simulink model "Pendulum_Native_1"  (R2021a)
settings: Solver=FixedStepDiscrete  StartTime=0.0  StopTime=inf  FixedStep=0.01  RelTol=1e-3
PostLoadFcn:
  | addpath(fileparts(get_param('Pendulum_Native_1','FileName')),fullfile(fileparts(get_param('Pendulum_Native_1','FileName')),'..','hardware'));
InitFcn:
  | addpath(fileparts(get_param('Pendulum_Native_1','FileName')),fullfile(fileparts(get_param('Pendulum_Native_1','FileName')),'..','hardware'));
libraries: sldrtlib x1
settings Model: Creator=YW  LastModifiedBy=YW
settings DataIOCC: SaveOutput=off  SignalLogging=off  SaveTime=off
settings DebuggingCC: AlgebraicLoopMsg=error

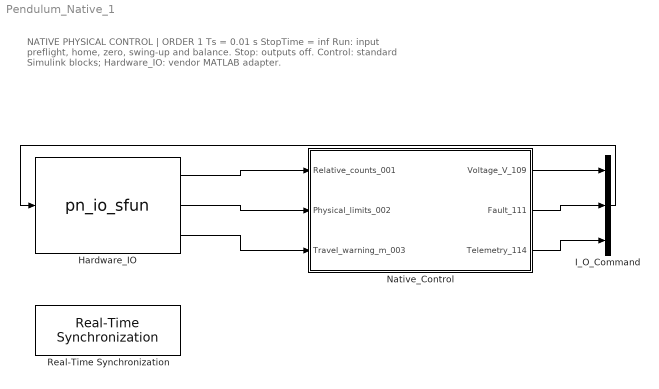
== system Pendulum_Native_1 ==
  note: NATIVE PHYSICAL CONTROL | ORDER 1
      | Ts = 0.01 s    StopTime = inf
      | Run: input preflight, home, zero, swing-up and balance. Stop: outputs off.
      | Control: standard Simulink blocks; Hardware_IO: vendor MATLAB adapter.
  Hardware_IO : M-S-Function  FunctionName=pn_io_sfun  Parameters=1
  I_O_Command : Mux  Inputs=3
  Native_Control : Subsystem
  Real-Time Synchronization : sldrtlib/Real-Time Synchronization  Priority=-100  SampleTime=0.01  MaxMissedTicks=1000000  ShowMissedTicks=off  YieldWhenWaiting=off
  wires:
  Hardware_IO/1 -> Native_Control/1(Relative_counts_001)
  Hardware_IO/2 -> Native_Control/2(Physical_limits_002)
  Hardware_IO/3 -> Native_Control/3(Travel_warning_m_003)
  Native_Control/1(Voltage_V_109) -> I_O_Command/1
  Native_Control/2(Fault_111) -> I_O_Command/2
  Native_Control/3(Telemetry_114) -> I_O_Command/3
  I_O_Command/1 -> Hardware_IO/1

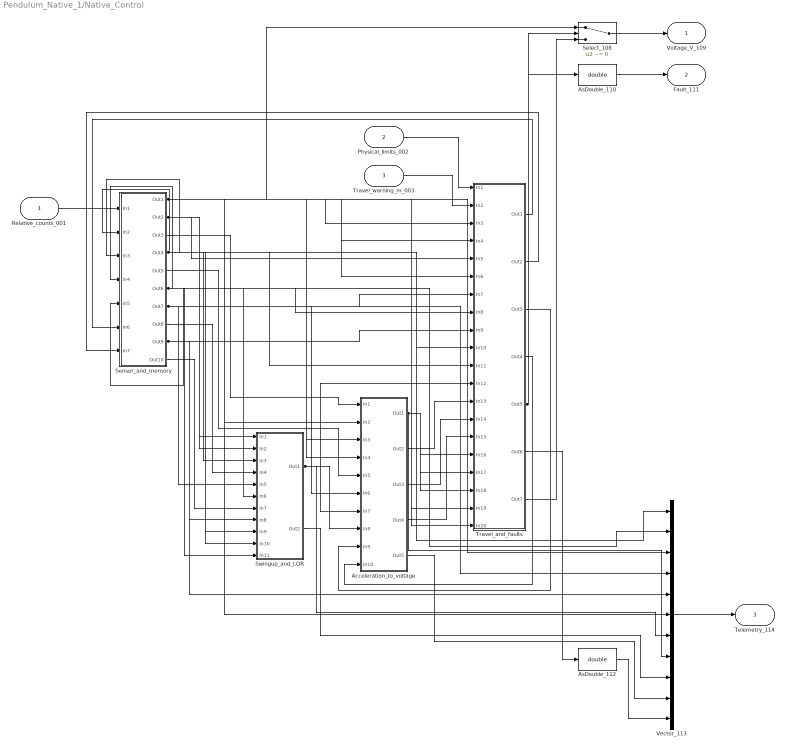
== system Pendulum_Native_1/Native_Control ==
  Relative_counts_001 : Inport  PortDimensions=2
  Physical_limits_002 : Inport  Port=2  PortDimensions=2
  Travel_warning_m_003 : Inport  Port=3  PortDimensions=1
  Acceleration_to_voltage : Subsystem
  AsDouble_110 : DataTypeConversion  OutDataTypeStr=double
  AsDouble_112 : DataTypeConversion  OutDataTypeStr=double
  Select_108 : Switch  Criteria=u2 ~= 0
  Sensor_and_memory : Subsystem
  Swingup_and_LQR : Subsystem
  Travel_and_faults : Subsystem
  Vector_113 : Mux  Inputs=11
  Voltage_V_109 : Outport
  Fault_111 : Outport  Port=2
  Telemetry_114 : Outport  Port=3
  wires:
  Travel_and_faults/4(Out4) -> Acceleration_to_voltage/10(In10)
  Vector_113/1 -> Telemetry_114/1
  Travel_and_faults/7(Out7) -> Select_108/3
  Travel_and_faults/3(Out3) -> Acceleration_to_voltage/9(In9)
  Travel_and_faults/6(Out6) -> AsDouble_112/1
  Travel_and_faults/2(Out2) -> Sensor_and_memory/7(In7)
  Travel_and_faults/1(Out1) -> Sensor_and_memory/6(In6)
  Sensor_and_memory/2(Out2) -> Travel_and_faults/5(In5), Swingup_and_LQR/1(In1), Swingup_and_LQR/2(In2)
  Acceleration_to_voltage/4(Out4) -> Travel_and_faults/15(In15)
  Select_108/1 -> Voltage_V_109/1
  Acceleration_to_voltage/3(Out3) -> Travel_and_faults/14(In14)
  Sensor_and_memory/5(Out5) -> Acceleration_to_voltage/5(In5)
  Acceleration_to_voltage/2(Out2) -> Travel_and_faults/13(In13)
  Sensor_and_memory/3(Out3) -> Acceleration_to_voltage/1(In1)
  Travel_warning_m_003/1 -> Travel_and_faults/2(In2)
  Sensor_and_memory/7(Out7) -> Vector_113/4, Acceleration_to_voltage/6(In6), Travel_and_faults/7(In7), Swingup_and_LQR/5(In5)
  Acceleration_to_voltage/1(Out1) -> Travel_and_faults/18(In18), Vector_113/8, Travel_and_faults/16(In16), Travel_and_faults/17(In17)
  Physical_limits_002/1 -> Travel_and_faults/1(In1)
  Acceleration_to_voltage/5(Out5) -> Vector_113/10
  Swingup_and_LQR/2(Out2) -> Vector_113/9
  Relative_counts_001/1 -> Sensor_and_memory/1(In1)
  Sensor_and_memory/10(Out10) -> Swingup_and_LQR/7(In7)
  Sensor_and_memory/8(Out8) -> Swingup_and_LQR/4(In4)
  AsDouble_112/1 -> Vector_113/11
  AsDouble_110/1 -> Fault_111/1
  Travel_and_faults/5(Out5) -> Select_108/2, AsDouble_110/1
  Swingup_and_LQR/1(Out1) -> Vector_113/7, Acceleration_to_voltage/7(In7), Acceleration_to_voltage/8(In8), Travel_and_faults/12(In12)
  Sensor_and_memory/1(Out1) -> Vector_113/3, Vector_113/6, Travel_and_faults/20(In20), Acceleration_to_voltage/3(In3), Select_108/1, Travel_and_faults/19(In19), Acceleration_to_voltage/4(In4), Travel_and_faults/6(In6), Acceleration_to_voltage/2(In2), Travel_and_faults/3(In3), Travel_and_faults/4(In4)
  Sensor_and_memory/4(Out4) -> Swingup_and_LQR/10(In10), Travel_and_faults/10(In10), Swingup_and_LQR/9(In9), Travel_and_faults/11(In11), Sensor_and_memory/3(In3), Vector_113/1, Sensor_and_memory/2(In2), Swingup_and_LQR/3(In3)
  Sensor_and_memory/6(Out6) -> Swingup_and_LQR/6(In6), Travel_and_faults/8(In8), Sensor_and_memory/4(In4), Swingup_and_LQR/11(In11), Vector_113/2, Sensor_and_memory/5(In5)
  Sensor_and_memory/9(Out9) -> Swingup_and_LQR/8(In8), Travel_and_faults/9(In9), Vector_113/5

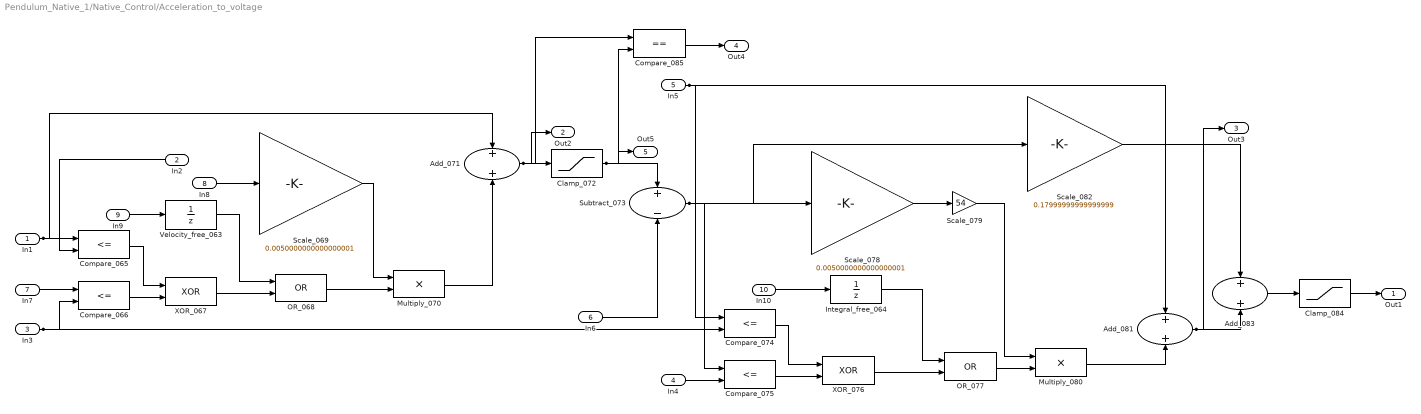
== system Pendulum_Native_1/Native_Control/Acceleration_to_voltage ==
  In1 : Inport
  In2 : Inport  Port=2
  In3 : Inport  Port=3
  In4 : Inport  Port=4
  In5 : Inport  Port=5
  In6 : Inport  Port=6
  In7 : Inport  Port=7
  In8 : Inport  Port=8
  In9 : Inport  Port=9
  In10 : Inport  Port=10
  Add_071 : Sum
  Add_081 : Sum
  Add_083 : Sum
  Clamp_072 : Saturate  UpperLimit=0.59999999999999998  LowerLimit=-0.59999999999999998
  Clamp_084 : Saturate  UpperLimit=1  LowerLimit=-1
  Compare_065 : RelationalOperator  Operator=<=  OutDataTypeStr=boolean  RndMeth=Simplest
  Compare_066 : RelationalOperator  Operator=<=  OutDataTypeStr=boolean  RndMeth=Simplest
  Compare_074 : RelationalOperator  Operator=<=  OutDataTypeStr=boolean  RndMeth=Simplest
  Compare_075 : RelationalOperator  Operator=<=  OutDataTypeStr=boolean  RndMeth=Simplest
  Compare_085 : RelationalOperator  Operator===  OutDataTypeStr=boolean  RndMeth=Simplest
  Integral_free_064 : UnitDelay  SampleTime=-1  HasFrameUpgradeWarning=on
  Multiply_070 : Product
  Multiply_080 : Product
  OR_068 : Logic  Operator=OR  AllPortsSameDT=off  OutDataTypeStr=boolean
  OR_077 : Logic  Operator=OR  AllPortsSameDT=off  OutDataTypeStr=boolean
  Scale_069 : Gain  Gain=0.0050000000000000001
  Scale_078 : Gain  Gain=0.0050000000000000001
  Scale_079 : Gain  Gain=54
  Scale_082 : Gain  Gain=0.17999999999999999
  Subtract_073 : Sum  Inputs=+-
  Velocity_free_063 : UnitDelay  SampleTime=-1  HasFrameUpgradeWarning=on
  XOR_067 : Logic  Operator=XOR  AllPortsSameDT=off  OutDataTypeStr=boolean
  XOR_076 : Logic  Operator=XOR  AllPortsSameDT=off  OutDataTypeStr=boolean
  Out1 : Outport
  Out2 : Outport  Port=2
  Out3 : Outport  Port=3
  Out4 : Outport  Port=4
  Out5 : Outport  Port=5
  wires:
  In6/1 -> Subtract_073/2
  In9/1 -> Velocity_free_063/1
  Compare_085/1 -> Out4/1
  In8/1 -> Scale_069/1
  In10/1 -> Integral_free_064/1
  Add_083/1 -> Clamp_084/1
  Scale_078/1 -> Scale_079/1
  Subtract_073/1 -> Compare_075/1, Scale_078/1, Scale_082/1
  OR_077/1 -> Multiply_080/2
  XOR_076/1 -> OR_077/2
  XOR_067/1 -> OR_068/2
  Scale_079/1 -> Multiply_080/1
  OR_068/1 -> Multiply_070/2
  In7/1 -> Compare_066/1
  In1/1 -> Add_071/1, Compare_065/1
  Compare_074/1 -> XOR_076/1
  Integral_free_064/1 -> OR_077/1
  Clamp_084/1 -> Out1/1
  Scale_069/1 -> Multiply_070/1
  Velocity_free_063/1 -> OR_068/1
  Multiply_070/1 -> Add_071/2
  Scale_082/1 -> Add_083/1
  Compare_066/1 -> XOR_067/2
  Multiply_080/1 -> Add_081/2
  Compare_075/1 -> XOR_076/2
  In2/1 -> Compare_065/2
  In4/1 -> Compare_075/2
  Compare_065/1 -> XOR_067/1
  Add_071/1 -> Compare_085/1, Out2/1, Clamp_072/1
  In3/1 -> Compare_066/2, Compare_074/2
  Clamp_072/1 -> Compare_085/2, Out5/1, Subtract_073/1
  Add_081/1 -> Add_083/2, Out3/1
  In5/1 -> Compare_074/1, Add_081/1

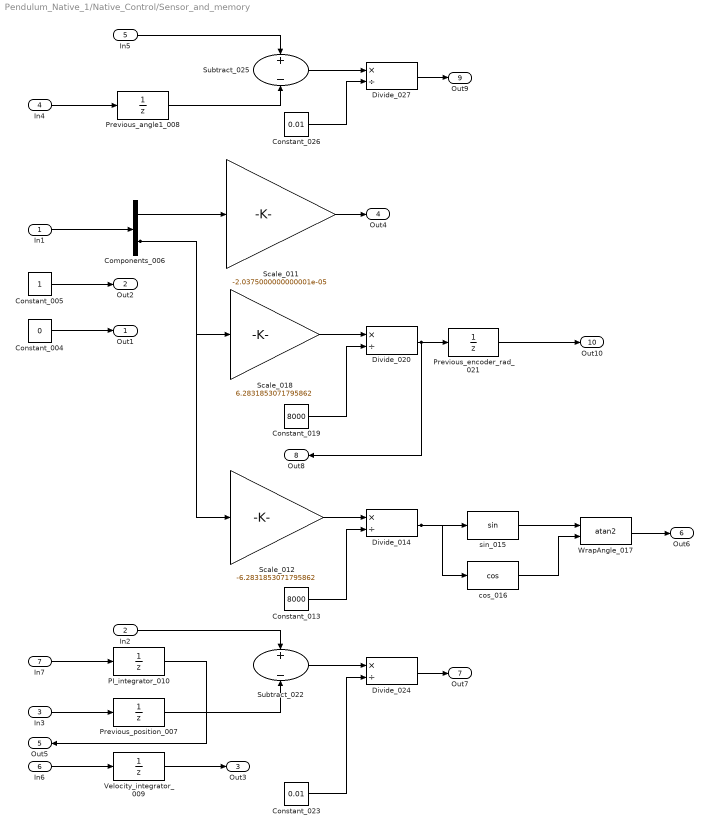
== system Pendulum_Native_1/Native_Control/Sensor_and_memory ==
  In1 : Inport
  In2 : Inport  Port=2
  In3 : Inport  Port=3
  In4 : Inport  Port=4
  In5 : Inport  Port=5
  In6 : Inport  Port=6
  In7 : Inport  Port=7
  Components_006 : Demux  Outputs=2
  Constant_004 : Constant  Value=0
  Constant_005 : Constant
  Constant_013 : Constant  Value=8000
  Constant_019 : Constant  Value=8000
  Constant_023 : Constant  Value=0.01
  Constant_026 : Constant  Value=0.01
  Divide_014 : Product  Inputs=*/
  Divide_020 : Product  Inputs=*/
  Divide_024 : Product  Inputs=*/
  Divide_027 : Product  Inputs=*/
  PI_integrator_010 : UnitDelay  SampleTime=-1  HasFrameUpgradeWarning=on
  Previous_angle1_008 : UnitDelay  SampleTime=-1  HasFrameUpgradeWarning=on
  Previous_encoder_rad_021 : UnitDelay  SampleTime=-1  HasFrameUpgradeWarning=on
  Previous_position_007 : UnitDelay  SampleTime=-1  HasFrameUpgradeWarning=on
  Scale_011 : Gain  Gain=-2.0375000000000001e-05
  Scale_012 : Gain  Gain=-6.2831853071795862
  Scale_018 : Gain  Gain=6.2831853071795862
  Subtract_022 : Sum  Inputs=+-
  Subtract_025 : Sum  Inputs=+-
  Velocity_integrator_009 : UnitDelay  SampleTime=-1  HasFrameUpgradeWarning=on
  WrapAngle_017 : Trigonometry  Operator=atan2
  cos_016 : Trigonometry  Operator=cos
  sin_015 : Trigonometry
  Out1 : Outport
  Out2 : Outport  Port=2
  Out3 : Outport  Port=3
  Out4 : Outport  Port=4
  Out5 : Outport  Port=5
  Out6 : Outport  Port=6
  Out7 : Outport  Port=7
  Out8 : Outport  Port=8
  Out9 : Outport  Port=9
  Out10 : Outport  Port=10
  wires:
  In5/1 -> Subtract_025/1
  In7/1 -> PI_integrator_010/1
  In4/1 -> Previous_angle1_008/1
  Scale_011/1 -> Out4/1
  PI_integrator_010/1 -> Out5/1
  Velocity_integrator_009/1 -> Out3/1
  Divide_024/1 -> Out7/1
  In3/1 -> Previous_position_007/1
  Divide_027/1 -> Out9/1
  Constant_004/1 -> Out1/1
  In1/1 -> Components_006/1
  Constant_026/1 -> Divide_027/2
  WrapAngle_017/1 -> Out6/1
  Scale_018/1 -> Divide_020/1
  Subtract_025/1 -> Divide_027/1
  In2/1 -> Subtract_022/1
  In6/1 -> Velocity_integrator_009/1
  Previous_position_007/1 -> Subtract_022/2
  Previous_encoder_rad_021/1 -> Out10/1
  Subtract_022/1 -> Divide_024/1
  Previous_angle1_008/1 -> Subtract_025/2
  Scale_012/1 -> Divide_014/1
  Constant_019/1 -> Divide_020/2
  sin_015/1 -> WrapAngle_017/1
  cos_016/1 -> WrapAngle_017/2
  Components_006/1 -> Scale_011/1
  Constant_023/1 -> Divide_024/2
  Constant_013/1 -> Divide_014/2
  Constant_005/1 -> Out2/1
  Divide_014/1 -> sin_015/1, cos_016/1
  Components_006/2 -> Scale_012/1, Scale_018/1
  Divide_020/1 -> Previous_encoder_rad_021/1, Out8/1

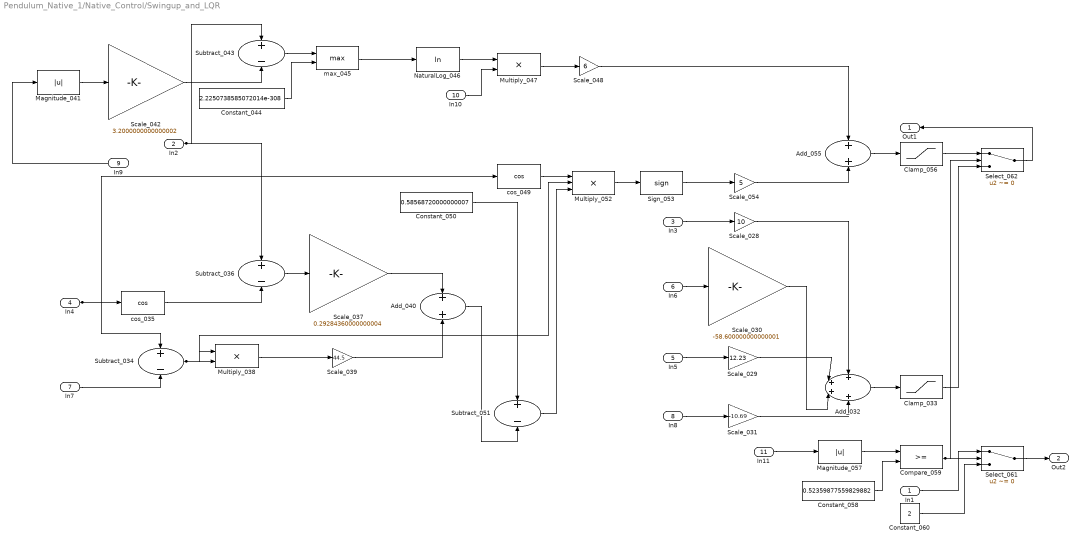
== system Pendulum_Native_1/Native_Control/Swingup_and_LQR ==
  In1 : Inport
  In2 : Inport  Port=2
  In3 : Inport  Port=3
  In4 : Inport  Port=4
  In5 : Inport  Port=5
  In6 : Inport  Port=6
  In7 : Inport  Port=7
  In8 : Inport  Port=8
  In9 : Inport  Port=9
  In10 : Inport  Port=10
  In11 : Inport  Port=11
  Add_032 : Sum  Inputs=++++
  Add_040 : Sum
  Add_055 : Sum
  Clamp_033 : Saturate  UpperLimit=10  LowerLimit=-10
  Clamp_056 : Saturate  UpperLimit=10  LowerLimit=-10
  Compare_059 : RelationalOperator  OutDataTypeStr=boolean  RndMeth=Simplest
  Constant_044 : Constant  Value=2.2250738585072014e-308
  Constant_050 : Constant  Value=0.58568720000000007
  Constant_058 : Constant  Value=0.52359877559829882
  Constant_060 : Constant  Value=2
  Magnitude_041 : Abs
  Magnitude_057 : Abs
  Multiply_038 : Product
  Multiply_047 : Product
  Multiply_052 : Product  Inputs=3
  NaturalLog_046 : Math  Operator=log  SaturateOnIntegerOverflow=on
  Scale_028 : Gain  Gain=10
  Scale_029 : Gain  Gain=12.23
  Scale_030 : Gain  Gain=-58.600000000000001
  Scale_031 : Gain  Gain=-10.69
  Scale_037 : Gain  Gain=0.29284360000000004
  Scale_039 : Gain  Gain=44.5
  Scale_042 : Gain  Gain=3.2000000000000002
  Scale_048 : Gain  Gain=6
  Scale_054 : Gain  Gain=5
  Select_061 : Switch  Criteria=u2 ~= 0
  Select_062 : Switch  Criteria=u2 ~= 0
  Sign_053 : Signum
  Subtract_034 : Sum  Inputs=+-
  Subtract_036 : Sum  Inputs=+-
  Subtract_043 : Sum  Inputs=+-
  Subtract_051 : Sum  Inputs=+-
  cos_035 : Trigonometry  Operator=cos
  cos_049 : Trigonometry  Operator=cos
  max_045 : MinMax  Function=max  Inputs=2
  Out1 : Outport
  Out2 : Outport  Port=2
  wires:
  In9/1 -> Magnitude_041/1
  Scale_054/1 -> Add_055/2
  In7/1 -> Subtract_034/2
  Select_062/1 -> Out1/1
  cos_049/1 -> Multiply_052/1
  Multiply_038/1 -> Scale_039/1
  Compare_059/1 -> Select_061/2, Select_062/2
  In10/1 -> Multiply_047/2
  In3/1 -> Scale_028/1
  In5/1 -> Scale_029/1
  Scale_029/1 -> Add_032/2
  In8/1 -> Scale_031/1
  In11/1 -> Magnitude_057/1
  NaturalLog_046/1 -> Multiply_047/1
  In6/1 -> Scale_030/1
  Multiply_047/1 -> Scale_048/1
  Subtract_043/1 -> max_045/1
  Sign_053/1 -> Scale_054/1
  Scale_028/1 -> Add_032/1
  Scale_042/1 -> Subtract_043/2
  Scale_039/1 -> Add_040/2
  Magnitude_057/1 -> Compare_059/1
  Magnitude_041/1 -> Scale_042/1
  Scale_031/1 -> Add_032/4
  Clamp_056/1 -> Select_062/1
  Constant_058/1 -> Compare_059/2
  Scale_037/1 -> Add_040/1
  Subtract_034/1 -> Multiply_038/2, Multiply_052/2, Multiply_038/1
  Scale_030/1 -> Add_032/3
  Add_032/1 -> Clamp_033/1
  Add_040/1 -> Subtract_051/2
  Subtract_036/1 -> Scale_037/1
  max_045/1 -> NaturalLog_046/1
  Add_055/1 -> Clamp_056/1
  Constant_050/1 -> Subtract_051/1
  Scale_048/1 -> Add_055/1
  Subtract_051/1 -> Multiply_052/3
  Constant_044/1 -> max_045/2
  Clamp_033/1 -> Select_062/3
  Constant_060/1 -> Select_061/3
  Multiply_052/1 -> Sign_053/1
  cos_035/1 -> Subtract_036/2
  In1/1 -> Select_061/1
  Select_061/1 -> Out2/1
  In2/1 -> Subtract_036/1, Subtract_043/1
  In4/1 -> cos_049/1, Subtract_034/1, cos_035/1

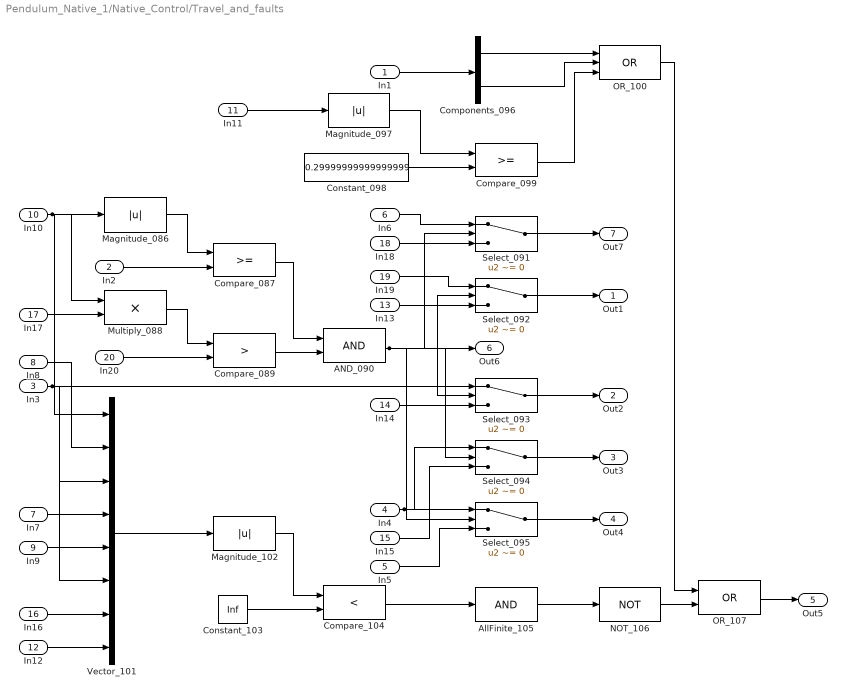
== system Pendulum_Native_1/Native_Control/Travel_and_faults ==
  In1 : Inport
  In2 : Inport  Port=2
  In3 : Inport  Port=3
  In4 : Inport  Port=4
  In5 : Inport  Port=5
  In6 : Inport  Port=6
  In7 : Inport  Port=7
  In8 : Inport  Port=8
  In9 : Inport  Port=9
  In10 : Inport  Port=10
  In11 : Inport  Port=11
  In12 : Inport  Port=12
  In13 : Inport  Port=13
  In14 : Inport  Port=14
  In15 : Inport  Port=15
  In16 : Inport  Port=16
  In17 : Inport  Port=17
  In18 : Inport  Port=18
  In19 : Inport  Port=19
  In20 : Inport  Port=20
  AND_090 : Logic  AllPortsSameDT=off  OutDataTypeStr=boolean
  AllFinite_105 : Logic  Inputs=1  AllPortsSameDT=off  OutDataTypeStr=boolean
  Compare_087 : RelationalOperator  OutDataTypeStr=boolean  RndMeth=Simplest
  Compare_089 : RelationalOperator  Operator=>  OutDataTypeStr=boolean  RndMeth=Simplest
  Compare_099 : RelationalOperator  OutDataTypeStr=boolean  RndMeth=Simplest
  Compare_104 : RelationalOperator  Operator=<  OutDataTypeStr=boolean  RndMeth=Simplest
  Components_096 : Demux  Outputs=2
  Constant_098 : Constant  Value=0.29999999999999999
  Constant_103 : Constant  Value=Inf
  Magnitude_086 : Abs
  Magnitude_097 : Abs
  Magnitude_102 : Abs
  Multiply_088 : Product
  NOT_106 : Logic  Operator=NOT  Inputs=1  AllPortsSameDT=off  OutDataTypeStr=boolean
  OR_100 : Logic  Operator=OR  Inputs=3  AllPortsSameDT=off  OutDataTypeStr=boolean
  OR_107 : Logic  Operator=OR  AllPortsSameDT=off  OutDataTypeStr=boolean
  Select_091 : Switch  Criteria=u2 ~= 0
  Select_092 : Switch  Criteria=u2 ~= 0
  Select_093 : Switch  Criteria=u2 ~= 0
  Select_094 : Switch  Criteria=u2 ~= 0
  Select_095 : Switch  Criteria=u2 ~= 0
  Vector_101 : Mux  Inputs=8
  Out1 : Outport
  Out2 : Outport  Port=2
  Out3 : Outport  Port=3
  Out4 : Outport  Port=4
  Out5 : Outport  Port=5
  Out6 : Outport  Port=6
  Out7 : Outport  Port=7
  wires:
  In8/1 -> Vector_101/2
  In20/1 -> Compare_089/2
  In2/1 -> Compare_087/2
  In16/1 -> Vector_101/7
  In7/1 -> Vector_101/4
  Constant_098/1 -> Compare_099/2
  In1/1 -> Components_096/1
  In17/1 -> Multiply_088/2
  Select_094/1 -> Out3/1
  In5/1 -> Select_095/3
  In15/1 -> Select_094/3
  Select_092/1 -> Out1/1
  In11/1 -> Magnitude_097/1
  Select_091/1 -> Out7/1
  Vector_101/1 -> Magnitude_102/1
  Constant_103/1 -> Compare_104/2
  AllFinite_105/1 -> NOT_106/1
  In9/1 -> Vector_101/5
  Components_096/1 -> OR_100/1
  Compare_099/1 -> OR_100/3
  In14/1 -> Select_093/3
  NOT_106/1 -> OR_107/2
  Magnitude_097/1 -> Compare_099/1
  In12/1 -> Vector_101/8
  Magnitude_086/1 -> Compare_087/1
  In13/1 -> Select_092/3
  Select_095/1 -> Out4/1
  In19/1 -> Select_092/1
  OR_100/1 -> OR_107/1
  Multiply_088/1 -> Compare_089/1
  Compare_104/1 -> AllFinite_105/1
  Compare_087/1 -> AND_090/1
  In18/1 -> Select_091/3
  OR_107/1 -> Out5/1
  In6/1 -> Select_091/1
  Compare_089/1 -> AND_090/2
  Magnitude_102/1 -> Compare_104/1
  AND_090/1 -> Select_094/2, Select_095/2, Select_093/2, Select_092/2, Select_091/2, Out6/1
  Components_096/2 -> OR_100/2
  Select_093/1 -> Out2/1
  In4/1 -> Select_094/1, Select_095/1
  In3/1 -> Vector_101/3, Vector_101/6, Select_093/1
  In10/1 -> Magnitude_086/1, Multiply_088/1, Vector_101/1
